simulink model "parrot_comm_host"  (R2024b)
settings: Solver=VariableStepAuto  StartTime=0.0  StopTime=inf  RelTol=1e-3
libraries: parrotlib x7
settings Model: Creator=keith  LastModifiedBy=keith

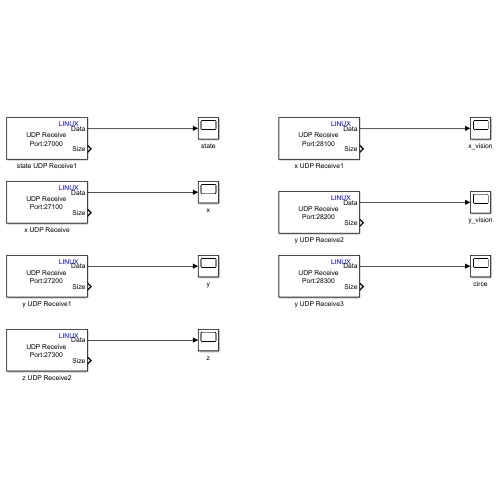
[thumbnail: Simulink's stored preview of the top-level diagram]
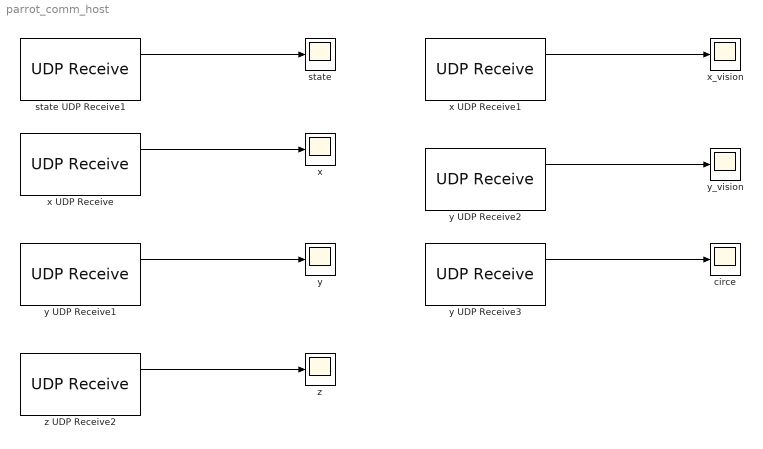
== system parrot_comm_host ==
  circe : Scope
  state : Scope
  state UDP Receive1 : parrotlib/UDP Receive  localURL='0.0.0.0'  localPort=27000  remoteURL='0.0.0.0'  remotePort=-1  recvBufferSize=8192  signalDatatype=double  dims=4  isVarSize=off  showBlockingTime=off  blockingTime=0  sampletime=0.005  blockPlatform=LINUX
  x : Scope
  x UDP Receive : parrotlib/UDP Receive  localURL='0.0.0.0'  localPort=27100  remoteURL='0.0.0.0'  remotePort=-1  recvBufferSize=8192  signalDatatype=single  dims=4  isVarSize=off  showBlockingTime=off  blockingTime=0  sampletime=0.005  blockPlatform=LINUX
  x UDP Receive1 : parrotlib/UDP Receive  localURL='0.0.0.0'  localPort=28100  remoteURL='0.0.0.0'  remotePort=-1  recvBufferSize=8192  signalDatatype=double  dims=4  isVarSize=off  showBlockingTime=off  blockingTime=0  sampletime=0.005  blockPlatform=LINUX
  x_vision : Scope
  y : Scope
  y UDP Receive1 : parrotlib/UDP Receive  localURL='0.0.0.0'  localPort=27200  remoteURL='0.0.0.0'  remotePort=-1  recvBufferSize=8192  signalDatatype=single  dims=4  isVarSize=off  showBlockingTime=off  blockingTime=0  sampletime=0.005  blockPlatform=LINUX
  y UDP Receive2 : parrotlib/UDP Receive  localURL='0.0.0.0'  localPort=28200  remoteURL='0.0.0.0'  remotePort=-1  recvBufferSize=8192  signalDatatype=double  dims=4  isVarSize=off  showBlockingTime=off  blockingTime=0  sampletime=0.005  blockPlatform=LINUX
  y UDP Receive3 : parrotlib/UDP Receive  localURL='0.0.0.0'  localPort=28300  remoteURL='0.0.0.0'  remotePort=-1  recvBufferSize=8192  signalDatatype=double  dims=4  isVarSize=off  showBlockingTime=off  blockingTime=0  sampletime=0.005  blockPlatform=LINUX
  y_vision : Scope
  z : Scope
  z UDP Receive2 : parrotlib/UDP Receive  localURL='0.0.0.0'  localPort=27300  remoteURL='0.0.0.0'  remotePort=-1  recvBufferSize=8192  signalDatatype=single  dims=4  isVarSize=off  showBlockingTime=off  blockingTime=0  sampletime=0.005  blockPlatform=LINUX
  wires:
  x UDP Receive/1 -> x/1
  z UDP Receive2/1 -> z/1
  y UDP Receive1/1 -> y/1
  state UDP Receive1/1 -> state/1
  x UDP Receive1/1 -> x_vision/1
  y UDP Receive2/1 -> y_vision/1
  y UDP Receive3/1 -> circe/1
